simulink model "Analyse_Modele_Complet_Initial"  (R2020b)
settings: Solver=VariableStepAuto  StartTime=0.0  StopTime=10.0  RelTol=1e-3
undefined symbols (not defined in the file or in its folder): A_complet, A_K1, B_complet, B_K1, C_complet, C_K1, D31, D32, D33, D_complet, D_K1
settings Model: Creator=Sandou  LastModifiedBy=Sandou

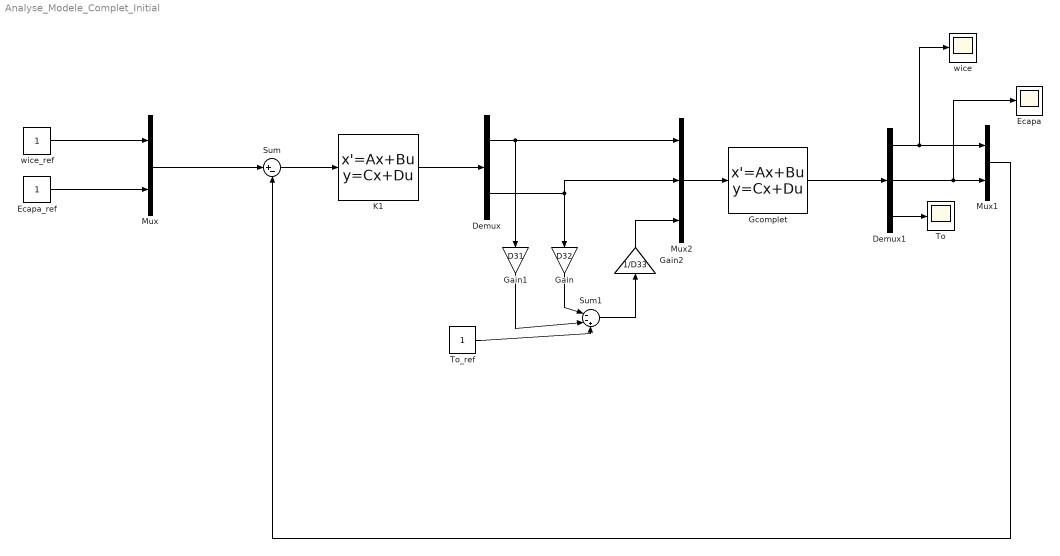
== system Analyse_Modele_Complet_Initial ==
  Demux : Demux  Outputs=2
  Demux1 : Demux  Outputs=3
  Ecapa : Scope
  Ecapa_ref : Constant
  Gain : Gain  Gain=D32
  Gain1 : Gain  Gain=D31
  Gain2 : Gain  Gain=1/D33
  Gcomplet : StateSpace  A=A_complet  B=B_complet  C=C_complet  D=D_complet  InitialCondition=0
  K1 : StateSpace  A=A_K1  B=B_K1  C=C_K1  D=D_K1  InitialCondition=0
  Mux : Mux  Inputs=2
  Mux1 : Mux  Inputs=2
  Mux2 : Mux  Inputs=3
  Sum : Sum  Inputs=|+-
  Sum1 : Sum  Inputs=|--+
  To : Scope
  To_ref : Constant
  wice : Scope
  wice_ref : Constant
  wires:
  Sum/1 -> K1/1
  Mux/1 -> Sum/1
  wice_ref/1 -> Mux/1
  Ecapa_ref/1 -> Mux/2
  K1/1 -> Demux/1
  Mux1/1 -> Sum/2
  Demux/2 -> Gain/1, Mux2/2
  Demux/1 -> Gain1/1, Mux2/1
  Mux2/1 -> Gcomplet/1
  Gcomplet/1 -> Demux1/1
  Demux1/1 -> wice/1, Mux1/1
  Demux1/2 -> Ecapa/1, Mux1/2
  Demux1/3 -> To/1
  Gain/1 -> Sum1/1
  Gain1/1 -> Sum1/2
  To_ref/1 -> Sum1/3
  Gain2/1 -> Mux2/3
  Sum1/1 -> Gain2/1
